simulink model "Localization_Ependorfv2"  (R2025a)
settings: Solver=VariableStepAuto  StartTime=0.0  StopTime=10.0  RelTol=1e-3
libraries: SignalEditorBlockLib x1
settings Model: Creator=Akash  LastModifiedBy=utkar
settings RTWCC: GPUComputeCapability=3.5

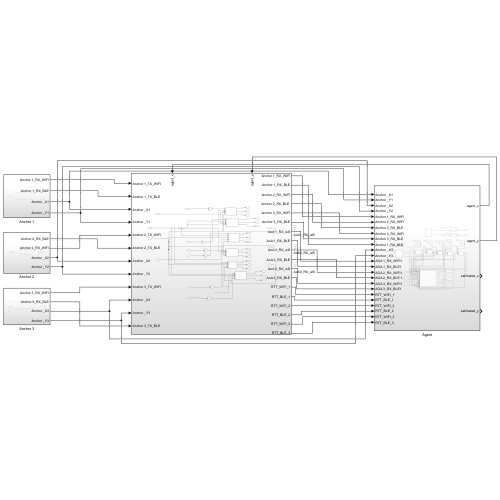
[thumbnail: Simulink's stored preview of the top-level diagram]
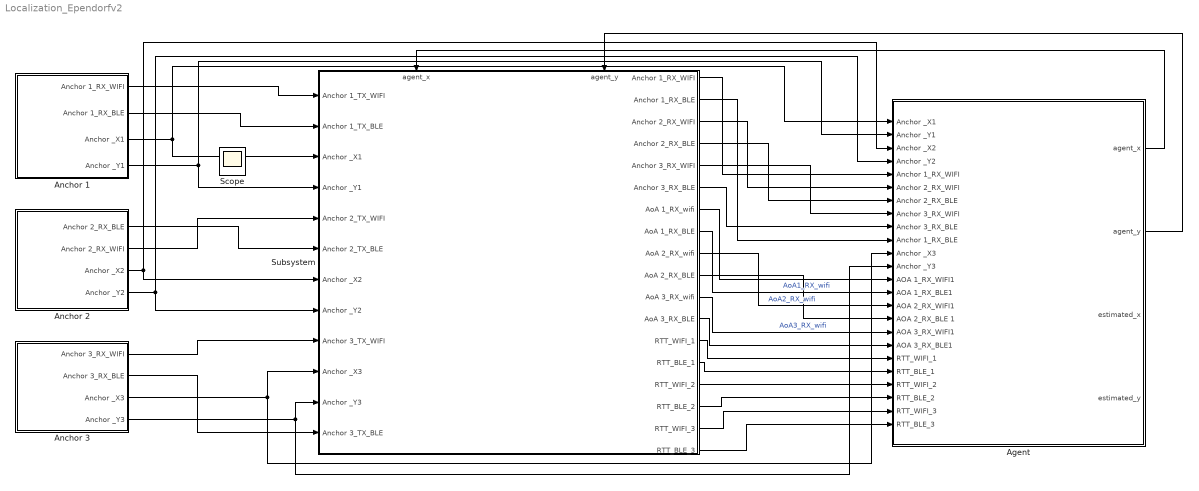
== system Localization_Ependorfv2 ==
  Agent : Subsystem
  Anchor 1 : Subsystem
  Anchor 2 : Subsystem
  Anchor 3 : Subsystem
  Subsystem : Subsystem
      settings: PortSchema="{\"entries\":[{\"content\":{\"sides\":[{\"content\":{\"connectorIds\":[\"In1\",\"In2\",\"In3\",\"In4\",\"In5\",\"In6\",\"In7\",\"In8\",\"In9\",\"In10\",\"In11\",\"In12\"]},\"type\":\"ConnectorPlacement.EquallySpacedRectSide\",\"uuid\":\"0405234f-5b8f-45a1-917e-93d58a1311a8\"},{\"content\":{\"connectorIds\":[\"Out1\",\"Out2\",\"Out3\",\"Out4\",\"Out5\",\"Out6\",\"Out7\",\"Out8\",\"Out9\",\"Out10\",\"Out11\",\"Out12\",\"Out13\",\"Out14\",\"Out15\",\"Out16\",\"Out17\",\"Out18\"],\"side\":\"RIGHT\"},\"type\":\"ConnectorPlacement.EquallySpacedRectSide\",\"uuid\":\"39d2f27a-3797-45c8-9e26-1762cabd752a\"},{\"content\":{\"connectorIds\":[\"In13\",\"In14\"],\"side\":\"TOP\"},\"type\":\"ConnectorPlacement.EquallySpacedRectSide\",\"uuid\":\"f6177108-a7d2-4d89-9cd9-46479219c011\"}]},\"type\":\"ConnectorPlacement.EquallySpacedConnector\",\"uuid\":\"e67eb188-6063-4e30-a59d-3af2b75346f2\"}],\"packageUris\":[\"http://schema.mathworks.com/mf0/Connector/R2020b\"],\"version\":\"1.0\"}"
  Scope : Scope
      settings: ActiveDisplayYMinimum=-0.44035255255063926  ActiveDisplayYMaximum=0.45352039029310781
  wires:
  Anchor 3/1(Anchor 3_RX_WIFI) -> Subsystem/9(Anchor 3_TX_WIFI)
  Anchor 3/2(Anchor 3_RX_BLE) -> Subsystem/12(Anchor 3_TX_BLE)
  Anchor 1/1(Anchor 1_RX_WIFI) -> Subsystem/1(Anchor 1_TX_WIFI)
  Anchor 1/2(Anchor 1_RX_BLE) -> Subsystem/2(Anchor 1_TX_BLE)
  Subsystem/1(Anchor 1_RX_WIFI) -> Agent/5(Anchor 1_RX_WIFI)
  Subsystem/2(Anchor 1_RX_BLE) -> Agent/10(Anchor 1_RX_BLE)
  Subsystem/3(Anchor 2_RX_WIFI) -> Agent/6(Anchor 2_RX_WIFI)
  Subsystem/4("Anchor 2_RX_BLE ") -> Agent/7("Anchor 2_RX_BLE ")
  Subsystem/5(Anchor 3_RX_WIFI) -> Agent/8(Anchor 3_RX_WIFI)
  Subsystem/6(Anchor 3_RX_BLE) -> Agent/9(Anchor 3_RX_BLE)
  Anchor 1/4(Anchor _Y1) -> Subsystem/4(Anchor _Y1), Agent/2(Anchor _Y1)
  Anchor 2/3(Anchor _X2) -> Agent/3(Anchor _X2), Subsystem/7(Anchor _X2)
  Anchor 2/4(Anchor _Y2) -> Agent/4(Anchor _Y2), Subsystem/8(Anchor _Y2)
  Anchor 3/3(Anchor _X3) -> Agent/11(Anchor _X3), Subsystem/10(Anchor _X3)
  Anchor 3/4(Anchor _Y3) -> Agent/12(Anchor _Y3), Subsystem/11(Anchor _Y3)
  Anchor 1/3(Anchor _X1) -> Subsystem/3(Anchor _X1), Agent/1(Anchor _X1)
  Agent/2(agent_y) -> Subsystem/14(agent_y)
  Agent/1(agent_x) -> Subsystem/13(agent_x)
  Subsystem/7(AoA 1_RX_wifi) -> Agent/13(AOA 1_RX_WIFI1)  "AoA1_RX_wifi"
  Subsystem/9(AoA 2_RX_wifi) -> Agent/15(AOA 2_RX_WIFI1)  "AoA2_RX_wifi"
  Subsystem/8(AoA 1_RX_BLE) -> Agent/14(AOA 1_RX_BLE1)
  Subsystem/10(AoA 2_RX_BLE) -> Agent/16(AOA 2_RX_BLE 1)
  Subsystem/11(AoA 3_RX_wifi) -> Agent/17(AOA 3_RX_WIFI1)  "AoA3_RX_wifi"
  Subsystem/12(AoA 3_RX_BLE) -> Agent/18(AOA 3_RX_BLE1)
  Subsystem/13(RTT_WIFI_1) -> Agent/19(RTT_WIFI_1)
  Subsystem/14(RTT_BLE_1) -> Agent/20(RTT_BLE_1)
  Subsystem/15(RTT_WIFI_2) -> Agent/21(RTT_WIFI_2)
  Subsystem/16(RTT_BLE_2) -> Agent/22(RTT_BLE_2)
  Subsystem/17(RTT_WIFI_3) -> Agent/23(RTT_WIFI_3)
  Subsystem/18(RTT_BLE_3) -> Agent/24(RTT_BLE_3)
  Anchor 2/1(Anchor 2_RX_BLE) -> Subsystem/6(Anchor 2_TX_BLE)
  Anchor 2/2(Anchor 2_RX_WIFI) -> Subsystem/5(Anchor 2_TX_WIFI)

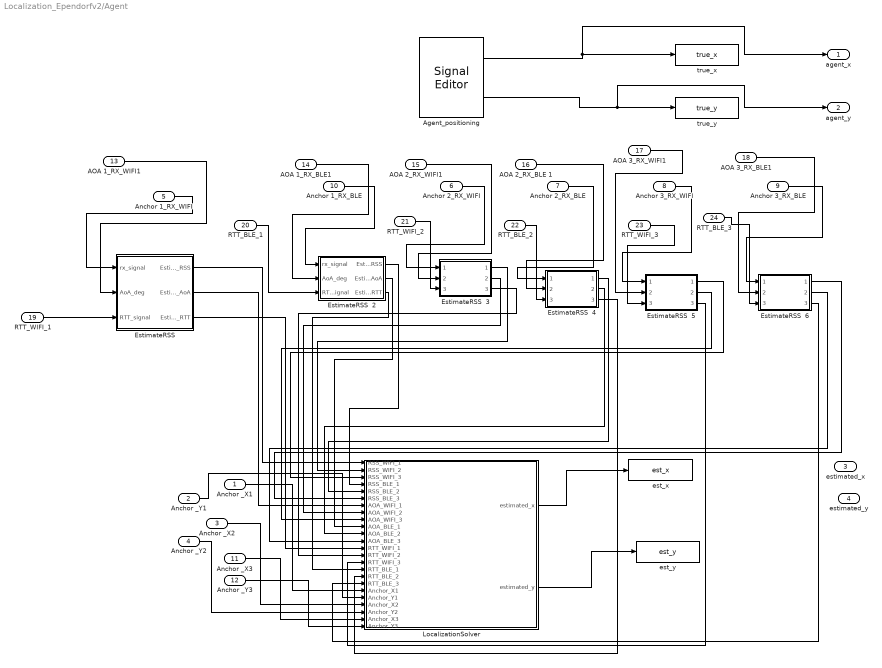
== system Localization_Ependorfv2/Agent ==
  Anchor _X1 : Inport
  Anchor _Y1 : Inport  Port=2
  Anchor _X2 : Inport  Port=3
  Anchor _Y2 : Inport  Port=4
  Anchor 1_RX_WIFI : Inport  Port=5
  Anchor 2_RX_WIFI : Inport  Port=6
  "Anchor 2_RX_BLE " : Inport  Port=7
  Anchor 3_RX_WIFI : Inport  Port=8
  Anchor 3_RX_BLE : Inport  Port=9
  Anchor 1_RX_BLE : Inport  Port=10
  Anchor _X3 : Inport  Port=11
  Anchor _Y3 : Inport  Port=12
  AOA 1_RX_WIFI1 : Inport  Port=13
  AOA 1_RX_BLE1 : Inport  Port=14
  AOA 2_RX_WIFI1 : Inport  Port=15
  AOA 2_RX_BLE 1 : Inport  Port=16
  AOA 3_RX_WIFI1 : Inport  Port=17
  AOA 3_RX_BLE1 : Inport  Port=18
  RTT_WIFI_1 : Inport  Port=19
  RTT_BLE_1 : Inport  Port=20
  RTT_WIFI_2 : Inport  Port=21
  RTT_BLE_2 : Inport  Port=22
  RTT_WIFI_3 : Inport  Port=23
  RTT_BLE_3 : Inport  Port=24
  Agent_positioning : SignalEditorBlockLib/Signal Editor  FileName=agent_path.mat  ActiveScenario=Scenario  ActiveSignal=Agent_x  IsBus=off  OutputBusObjectStr=Bus: BusObject  SampleTime=0  Interpolate=off  ZeroCross=off  OutputAfterFinalValue=Setting to zero  Unit=inherit  PreserveSignalName=on  ApplySigPropsToAllScenarios=on  ApplySigPropsToAllSignals=off  SignalPropertySource=Dialog parameters
  "EstimateRSS " : MATLAB Function  TreatAsAtomicUnit=on
  EstimateRSS  2 : MATLAB Function  TreatAsAtomicUnit=on
  EstimateRSS  3 : MATLAB Function  TreatAsAtomicUnit=on
  EstimateRSS  4 : MATLAB Function  TreatAsAtomicUnit=on
  EstimateRSS  5 : MATLAB Function  TreatAsAtomicUnit=on
  EstimateRSS  6 : MATLAB Function  TreatAsAtomicUnit=on
  LocalizationSolver : MATLAB Function  TreatAsAtomicUnit=on
  est_x : ToWorkspace  VariableName=est_x  SampleTime=-1
  est_y : ToWorkspace  VariableName=est_y  SampleTime=-1
  true_x : ToWorkspace  VariableName=true_x  SampleTime=-1
  true_y : ToWorkspace  VariableName=true_y  SampleTime=-1
  agent_x : Outport
  agent_y : Outport  Port=2
  estimated_x : Outport  Port=3
  estimated_y : Outport  Port=4
  wires:
  LocalizationSolver/2(estimated_y) -> est_y/1
  Anchor 2_RX_WIFI/1 -> EstimateRSS  3/1(rx_signal)
  Anchor 1_RX_BLE/1 -> EstimateRSS  2/1(rx_signal)
  "Anchor 2_RX_BLE "/1 -> EstimateRSS  4/1(rx_signal)
  Anchor 3_RX_WIFI/1 -> EstimateRSS  5/1(rx_signal)
  Anchor 3_RX_BLE/1 -> EstimateRSS  6/1(rx_signal)
  Agent_positioning/1 -> agent_x/1, true_x/1
  Agent_positioning/2 -> agent_y/1, true_y/1
  LocalizationSolver/1(estimated_x) -> est_x/1
  Anchor 1_RX_WIFI/1 -> "EstimateRSS "/1(rx_signal)
  AOA 1_RX_WIFI1/1 -> "EstimateRSS "/2(AoA_deg)
  AOA 1_RX_BLE1/1 -> EstimateRSS  2/2(AoA_deg)
  AOA 2_RX_WIFI1/1 -> EstimateRSS  3/2(AoA_deg)
  AOA 2_RX_BLE 1/1 -> EstimateRSS  4/2(AoA_deg)
  AOA 3_RX_WIFI1/1 -> EstimateRSS  5/2(AoA_deg)
  AOA 3_RX_BLE1/1 -> EstimateRSS  6/2(AoA_deg)
  Anchor _Y3/1 -> LocalizationSolver/24(Anchor_Y3)
  Anchor _X3/1 -> LocalizationSolver/23(Anchor_X3)
  Anchor _Y2/1 -> LocalizationSolver/22(Anchor_Y2)
  Anchor _X2/1 -> LocalizationSolver/21(Anchor_X2)
  Anchor _Y1/1 -> LocalizationSolver/20(Anchor_Y1)
  Anchor _X1/1 -> LocalizationSolver/19(Anchor_X1)
  "EstimateRSS "/1(Estimated_RSS) -> LocalizationSolver/1(RSS_WIFI_1)
  EstimateRSS  3/1(Estimated_RSS) -> LocalizationSolver/2(RSS_WIFI_2)
  EstimateRSS  5/1(Estimated_RSS) -> LocalizationSolver/3(RSS_WIFI_3)
  EstimateRSS  2/1(Estimated_RSS) -> LocalizationSolver/4(RSS_BLE_1)
  EstimateRSS  4/1(Estimated_RSS) -> LocalizationSolver/5(RSS_BLE_2)
  EstimateRSS  6/1(Estimated_RSS) -> LocalizationSolver/6(RSS_BLE_3)
  "EstimateRSS "/2(Estimated_AoA) -> LocalizationSolver/7(AOA_WIFI_1)
  EstimateRSS  3/2(Estimated_AoA) -> LocalizationSolver/8(AOA_WIFI_2)
  EstimateRSS  5/2(Estimated_AoA) -> LocalizationSolver/9(AOA_WIFI_3)
  EstimateRSS  2/2(Estimated_AoA) -> LocalizationSolver/10(AOA_BLE_1)
  EstimateRSS  4/2(Estimated_AoA) -> LocalizationSolver/11(AOA_BLE_2)
  EstimateRSS  6/2(Estimated_AoA) -> LocalizationSolver/12(AOA_BLE_3)
  RTT_WIFI_1/1 -> "EstimateRSS "/3(RTT_signal)
  RTT_BLE_1/1 -> EstimateRSS  2/3(RTT_signal)
  RTT_WIFI_2/1 -> EstimateRSS  3/3(RTT_signal)
  RTT_BLE_2/1 -> EstimateRSS  4/3(RTT_signal)
  RTT_WIFI_3/1 -> EstimateRSS  5/3(RTT_signal)
  RTT_BLE_3/1 -> EstimateRSS  6/3(RTT_signal)
  "EstimateRSS "/3(Estimated_RTT) -> LocalizationSolver/13(RTT_WIFI_1)
  EstimateRSS  2/3(Estimated_RTT) -> LocalizationSolver/16(RTT_BLE_1)
  EstimateRSS  3/3(Estimated_RTT) -> LocalizationSolver/14(RTT_WIFI_2)
  EstimateRSS  4/3(Estimated_RTT) -> LocalizationSolver/17(RTT_BLE_2)
  EstimateRSS  5/3(Estimated_RTT) -> LocalizationSolver/15(RTT_WIFI_3)
  EstimateRSS  6/3(Estimated_RTT) -> LocalizationSolver/18(RTT_BLE_3)

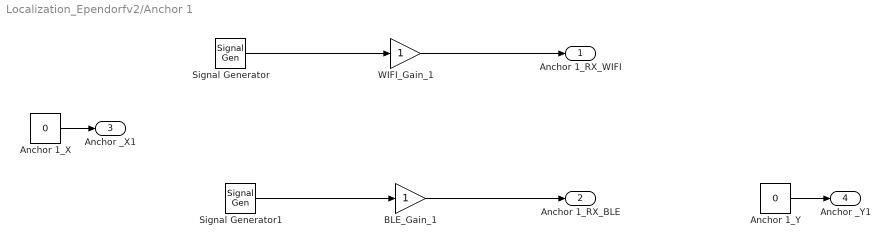
== system Localization_Ependorfv2/Anchor 1 ==
  Anchor 1_X : Constant  Value=0
  Anchor 1_Y : Constant  Value=0
  BLE_Gain_1 : Gain
  Signal Generator : SignalGenerator  Amplitude=10  Units=rad/sec
  Signal Generator1 : SignalGenerator  Amplitude=10  Units=rad/sec
  WIFI_Gain_1 : Gain
  Anchor 1_RX_WIFI : Outport
  Anchor 1_RX_BLE : Outport  Port=2
  Anchor _X1 : Outport  Port=3
  Anchor _Y1 : Outport  Port=4
  wires:
  Signal Generator/1 -> WIFI_Gain_1/1
  Signal Generator1/1 -> BLE_Gain_1/1
  Anchor 1_X/1 -> Anchor _X1/1
  Anchor 1_Y/1 -> Anchor _Y1/1
  WIFI_Gain_1/1 -> Anchor 1_RX_WIFI/1
  BLE_Gain_1/1 -> Anchor 1_RX_BLE/1

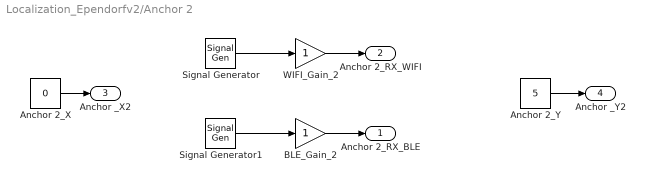
== system Localization_Ependorfv2/Anchor 2 ==
  Anchor 2_X : Constant  Value=0
  Anchor 2_Y : Constant  Value=5
  BLE_Gain_2 : Gain
  Signal Generator : SignalGenerator  Amplitude=10  Units=rad/sec
  Signal Generator1 : SignalGenerator  Amplitude=10  Units=rad/sec
  WIFI_Gain_2 : Gain
  Anchor 2_RX_BLE : Outport
  Anchor 2_RX_WIFI : Outport  Port=2
  Anchor _X2 : Outport  Port=3
  Anchor _Y2 : Outport  Port=4
  wires:
  Signal Generator1/1 -> BLE_Gain_2/1
  Signal Generator/1 -> WIFI_Gain_2/1
  Anchor 2_X/1 -> Anchor _X2/1
  Anchor 2_Y/1 -> Anchor _Y2/1
  WIFI_Gain_2/1 -> Anchor 2_RX_WIFI/1
  BLE_Gain_2/1 -> Anchor 2_RX_BLE/1

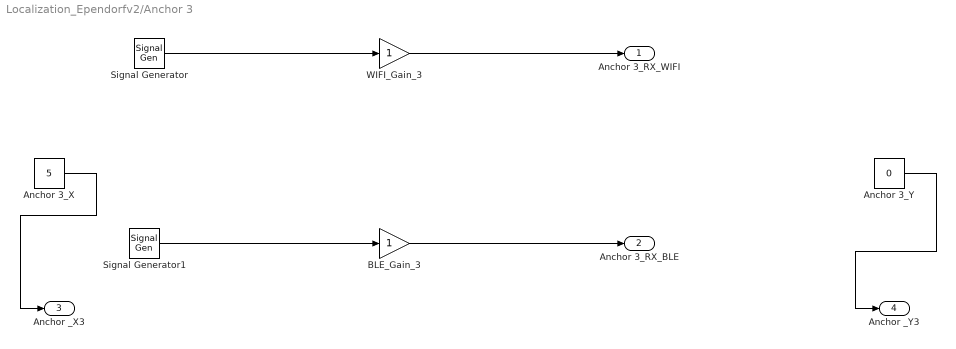
== system Localization_Ependorfv2/Anchor 3 ==
  Anchor 3_X : Constant  Value=5
  Anchor 3_Y : Constant  Value=0
  BLE_Gain_3 : Gain
  Signal Generator : SignalGenerator  Amplitude=10  Units=rad/sec
  Signal Generator1 : SignalGenerator  Amplitude=10  Units=rad/sec
  WIFI_Gain_3 : Gain
  Anchor 3_RX_WIFI : Outport
  Anchor 3_RX_BLE : Outport  Port=2
  Anchor _X3 : Outport  Port=3
  Anchor _Y3 : Outport  Port=4
  wires:
  Signal Generator1/1 -> BLE_Gain_3/1
  Signal Generator/1 -> WIFI_Gain_3/1
  Anchor 3_X/1 -> Anchor _X3/1
  Anchor 3_Y/1 -> Anchor _Y3/1
  WIFI_Gain_3/1 -> Anchor 3_RX_WIFI/1
  BLE_Gain_3/1 -> Anchor 3_RX_BLE/1

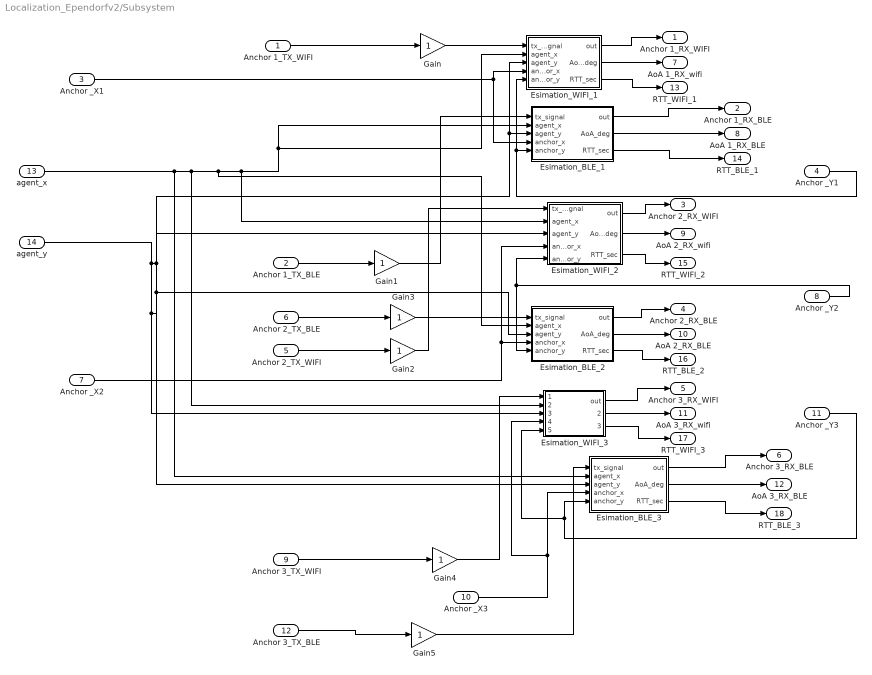
== system Localization_Ependorfv2/Subsystem ==
  Anchor 1_TX_WIFI : Inport
  Anchor 1_TX_BLE : Inport  Port=2
  Anchor _X1 : Inport  Port=3
  Anchor _Y1 : Inport  Port=4
  Anchor 2_TX_WIFI : Inport  Port=5
  Anchor 2_TX_BLE : Inport  Port=6
  Anchor _X2 : Inport  Port=7
  Anchor _Y2 : Inport  Port=8
  Anchor 3_TX_WIFI : Inport  Port=9
  Anchor _X3 : Inport  Port=10
  Anchor _Y3 : Inport  Port=11
  Anchor 3_TX_BLE : Inport  Port=12
  agent_x : Inport  Port=13
  agent_y : Inport  Port=14
  Esimation_BLE_1 : MATLAB Function  TreatAsAtomicUnit=on
  Esimation_BLE_2 : MATLAB Function  TreatAsAtomicUnit=on
  Esimation_BLE_3 : MATLAB Function  TreatAsAtomicUnit=on
  "Esimation_WIFI_1 " : MATLAB Function  TreatAsAtomicUnit=on
  Esimation_WIFI_2 : MATLAB Function  TreatAsAtomicUnit=on
  Esimation_WIFI_3 : MATLAB Function  TreatAsAtomicUnit=on
  Gain{,1..5} (6 alike) : Gain
  Anchor 1_RX_WIFI : Outport
  Anchor 1_RX_BLE : Outport  Port=2
  Anchor 2_RX_WIFI : Outport  Port=3
  "Anchor 2_RX_BLE " : Outport  Port=4
  Anchor 3_RX_WIFI : Outport  Port=5
  Anchor 3_RX_BLE : Outport  Port=6
  AoA 1_RX_wifi : Outport  Port=7
  AoA 1_RX_BLE : Outport  Port=8
  AoA 2_RX_wifi : Outport  Port=9
  AoA 2_RX_BLE : Outport  Port=10
  AoA 3_RX_wifi : Outport  Port=11
  AoA 3_RX_BLE : Outport  Port=12
  RTT_WIFI_1 : Outport  Port=13
  RTT_BLE_1 : Outport  Port=14
  RTT_WIFI_2 : Outport  Port=15
  RTT_BLE_2 : Outport  Port=16
  RTT_WIFI_3 : Outport  Port=17
  RTT_BLE_3 : Outport  Port=18
  wires:
  Anchor 1_TX_WIFI/1 -> Gain/1
  Anchor 1_TX_BLE/1 -> Gain1/1
  Anchor 2_TX_WIFI/1 -> Gain2/1
  Anchor 2_TX_BLE/1 -> Gain3/1
  Anchor 3_TX_WIFI/1 -> Gain4/1
  Anchor 3_TX_BLE/1 -> Gain5/1
  "Esimation_WIFI_1 "/1(out) -> Anchor 1_RX_WIFI/1
  Esimation_BLE_1/1(out) -> Anchor 1_RX_BLE/1
  Esimation_WIFI_2/1(out) -> Anchor 2_RX_WIFI/1
  Esimation_BLE_2/1(out) -> "Anchor 2_RX_BLE "/1
  Esimation_WIFI_3/1(out) -> Anchor 3_RX_WIFI/1
  Esimation_BLE_3/1(out) -> Anchor 3_RX_BLE/1
  Anchor _X3/1 -> Esimation_BLE_3/4(anchor_x), Esimation_WIFI_3/4(anchor_x)
  Gain/1 -> "Esimation_WIFI_1 "/1(tx_signal)
  Gain1/1 -> Esimation_BLE_1/1(tx_signal)
  Gain2/1 -> Esimation_WIFI_2/1(tx_signal)
  Gain3/1 -> Esimation_BLE_2/1(tx_signal)
  Gain4/1 -> Esimation_WIFI_3/1(tx_signal)
  Gain5/1 -> Esimation_BLE_3/1(tx_signal)
  Esimation_BLE_3/2(AoA_deg) -> AoA 3_RX_BLE/1
  Esimation_WIFI_3/2(AoA_deg) -> AoA 3_RX_wifi/1
  Esimation_BLE_2/2(AoA_deg) -> AoA 2_RX_BLE/1
  Esimation_WIFI_2/2(AoA_deg) -> AoA 2_RX_wifi/1
  Esimation_BLE_1/2(AoA_deg) -> AoA 1_RX_BLE/1
  "Esimation_WIFI_1 "/2(AoA_deg) -> AoA 1_RX_wifi/1
  agent_x/1 -> Esimation_BLE_1/2(agent_x), "Esimation_WIFI_1 "/2(agent_x), Esimation_WIFI_2/2(agent_x), Esimation_BLE_2/2(agent_x), Esimation_WIFI_3/2(agent_x), Esimation_BLE_3/2(agent_x)
  agent_y/1 -> Esimation_WIFI_3/3(agent_y), Esimation_BLE_2/3(agent_y), Esimation_WIFI_2/3(agent_y), Esimation_BLE_3/3(agent_y), Esimation_BLE_1/3(agent_y), "Esimation_WIFI_1 "/3(agent_y)
  Anchor _X1/1 -> Esimation_BLE_1/4(anchor_x), "Esimation_WIFI_1 "/4(anchor_x)
  Anchor _Y1/1 -> "Esimation_WIFI_1 "/5(anchor_y), Esimation_BLE_1/5(anchor_y)
  Anchor _X2/1 -> Esimation_BLE_2/4(anchor_x), Esimation_WIFI_2/4(anchor_x)
  Anchor _Y2/1 -> Esimation_BLE_2/5(anchor_y), Esimation_WIFI_2/5(anchor_y)
  Anchor _Y3/1 -> Esimation_WIFI_3/5(anchor_y), Esimation_BLE_3/5(anchor_y)
  "Esimation_WIFI_1 "/3(RTT_sec) -> RTT_WIFI_1/1
  Esimation_BLE_1/3(RTT_sec) -> RTT_BLE_1/1
  Esimation_WIFI_2/3(RTT_sec) -> RTT_WIFI_2/1
  Esimation_BLE_2/3(RTT_sec) -> RTT_BLE_2/1
  Esimation_WIFI_3/3(RTT_sec) -> RTT_WIFI_3/1
  Esimation_BLE_3/3(RTT_sec) -> RTT_BLE_3/1

== matlab function Localization_Ependorfv2/Subsystem/Esimation_BLE_2 ==
  data: tx_signal input; agent_x input; out output; agent_y input; anchor_x input; anchor_y input; AoA_deg output; RTT_sec output
function [out, AoA_deg, RTT_sec] = applyPathLossWithAOA_BLE(tx_signal, agent_x, agent_y, anchor_x, anchor_y)
% applyPathLossWithAOA_BLE: Simulates signal attenuation, AoA, and RTT for BLE

% === 1. Compute Distance ===
d = sqrt((agent_x - anchor_x)^2 + (agent_y - anchor_y)^2);
d0 = 1;
d = max(d, d0);

% === 2. Path Loss Model (BLE)
Ptx = 0;       
PL0 = 50;      % BLE generally has higher base loss
n   = 3;       % Stronger attenuation indoors for BLE
PL  = PL0 + 10 * n * log10(d / d0);

% === 3. Attenuate Signal ===
attenuation = 10.^(-PL / 20);  
out = tx_signal * attenuation;

% === 4. AoA Calculation (BLE - slightly noisier)
aoa_noise_std_deg = 5;
dx = agent_x - anchor_x;
dy = agent_y - anchor_y;
AoA_rad = atan2(dy, dx);
AoA_rad_noisy = AoA_rad + deg2rad(randn * aoa_noise_std_deg);
AoA_deg = mod(rad2deg(AoA_rad_noisy), 360);

% === 5. Simulate RTT (BLE less accurate: ~5 ns noise)
c = 3e8;  
rtt_noise_std = 5e-9;  
RTT_sec = 2 * d / c + randn * rtt_noise_std;

end

== matlab function Localization_Ependorfv2/Subsystem/Esimation_WIFI_3 ==
  data: tx_signal input; agent_x input; out output; agent_y input; anchor_x input; anchor_y input; AoA_deg output; RTT_sec output
function [out, AoA_deg, RTT_sec] = applyPathLossWithAOA_WiFi(tx_signal, agent_x, agent_y, anchor_x, anchor_y)
% applyPathLossWithAOA_WiFi: Simulates signal attenuation, AoA, and RTT for WiFi

% === 1. Compute Distance ===
d = sqrt((agent_x - anchor_x)^2 + (agent_y - anchor_y)^2);
d0 = 1;
d = max(d, d0);

% === 2. Path Loss Model (WiFi) ===
Ptx = 0;       % dBm
PL0 = 30;      % Reference loss at 1m (WiFi)
n   = 2.2;     % Path loss exponent for indoor WiFi
PL  = PL0 + 10 * n * log10(d / d0);

% === 3. Attenuate Signal ===
attenuation = 10.^(-PL / 20);  
out = tx_signal * attenuation;

% === 4. AoA Calculation (WiFi - lower noise)
aoa_noise_std_deg = 2;
dx = agent_x - anchor_x;
dy = agent_y - anchor_y;
AoA_rad = atan2(dy, dx);
AoA_rad_noisy = AoA_rad + deg2rad(randn * aoa_noise_std_deg);
AoA_deg = mod(rad2deg(AoA_rad_noisy), 360);

% === 5. Simulate RTT (WiFi typically accurate to ~1 ns)
c = 3e8;  
rtt_noise_std = 1e-9;  
RTT_sec = 2 * d / c + randn * rtt_noise_std;

end

== matlab function Localization_Ependorfv2/Subsystem/Esimation_BLE_3 ==
  data: tx_signal input; agent_x input; agent_y input; out output; anchor_x input; anchor_y input; AoA_deg output; RTT_sec output
function [out, AoA_deg, RTT_sec] = applyPathLossWithAOA_BLE(tx_signal, agent_x, agent_y, anchor_x, anchor_y)
% applyPathLossWithAOA_BLE: Simulates signal attenuation, AoA, and RTT for BLE

% === 1. Compute Distance ===
d = sqrt((agent_x - anchor_x)^2 + (agent_y - anchor_y)^2);
d0 = 1;
d = max(d, d0);

% === 2. Path Loss Model (BLE)
Ptx = 0;       
PL0 = 50;      % BLE generally has higher base loss
n   = 3;       % Stronger attenuation indoors for BLE
PL  = PL0 + 10 * n * log10(d / d0);

% === 3. Attenuate Signal ===
attenuation = 10.^(-PL / 20);  
out = tx_signal * attenuation;

% === 4. AoA Calculation (BLE - slightly noisier)
aoa_noise_std_deg = 5;
dx = agent_x - anchor_x;
dy = agent_y - anchor_y;
AoA_rad = atan2(dy, dx);
AoA_rad_noisy = AoA_rad + deg2rad(randn * aoa_noise_std_deg);
AoA_deg = mod(rad2deg(AoA_rad_noisy), 360);

% === 5. Simulate RTT (BLE less accurate: ~5 ns noise)
c = 3e8;  
rtt_noise_std = 5e-9;  
RTT_sec = 2 * d / c + randn * rtt_noise_std;

end

== matlab function Localization_Ependorfv2/Agent/LocalizationSolver ==
  data: RSS_WIFI_1 input; RSS_WIFI_2 input; RSS_WIFI_3 input; estimated_x output double size=1; estimated_y output double size=1; RSS_BLE_1 input double size=1; RSS_BLE_2 input double size=1; RSS_BLE_3 input; AOA_WIFI_1 input; AOA_WIFI_2 input; AOA_WIFI_3 input; AOA_BLE_1 input; AOA_BLE_2 input; AOA_BLE_3 input; RTT_WIFI_1 input; RTT_WIFI_2 input; RTT_WIFI_3 input; RTT_BLE_1 input; RTT_BLE_2 input; RTT_BLE_3 input; Anchor_X1 input double size=1; Anchor_Y1 input double size=1; Anchor_X2 input double size=1; Anchor_Y2 input double size=1; Anchor_X3 input double size=1; Anchor_Y3 input double size=1
function [estimated_x, estimated_y] = fcn( ...
    RSS_WIFI_1, RSS_WIFI_2, RSS_WIFI_3, ...
    RSS_BLE_1,  RSS_BLE_2,  RSS_BLE_3, ...
    AOA_WIFI_1, AOA_WIFI_2, AOA_WIFI_3, ...
    AOA_BLE_1,  AOA_BLE_2,  AOA_BLE_3, ...
    RTT_WIFI_1, RTT_WIFI_2, RTT_WIFI_3, ...
    RTT_BLE_1,  RTT_BLE_2,  RTT_BLE_3, ...
    Anchor_X1, Anchor_Y1, ...
    Anchor_X2, Anchor_Y2, ...
    Anchor_X3, Anchor_Y3)

% === 1. Collect RSS measurements ===
RSS_wifi = [RSS_WIFI_1; RSS_WIFI_2; RSS_WIFI_3];
RSS_ble  = [RSS_BLE_1;  RSS_BLE_2;  RSS_BLE_3];
RSS_all  = [RSS_wifi; RSS_ble];

% === 2. Anchor positions duplicated for BLE ===
anchors_x = [Anchor_X1; Anchor_X2; Anchor_X3];
anchors_y = [Anchor_Y1; Anchor_Y2; Anchor_Y3];
anchors_x_all = [anchors_x; anchors_x];  % Wi-Fi + BLE
anchors_y_all = [anchors_y; anchors_y];

% === 3. Convert RSS to distance ===
Pt  = 0;    % Transmit power [dBm]
PL0 = 44;   % Path loss at 1m [dB]
n   = 1.9;  % Path loss exponent
d0  = 1;    % reference distance [m]

estimated_d_rss = d0 * 10.^((Pt - PL0 - RSS_all) ./ (10 * n));
estimated_d_rss = min(estimated_d_rss, 100); % cap large distances

% === 4. Combine all AoA angles ===
aoa_angles_deg = [AOA_WIFI_1; AOA_WIFI_2; AOA_WIFI_3; ...
                  AOA_BLE_1;  AOA_BLE_2;  AOA_BLE_3];

% === 5. RTT-based Distance Estimation ===
c = 3e8;  % speed of light [m/s]
RTT_all = [RTT_WIFI_1; RTT_WIFI_2; RTT_WIFI_3; ...
           RTT_BLE_1;  RTT_BLE_2;  RTT_BLE_3];
estimated_d_rtt = RTT_all * c / 2;
estimated_d_rtt = min(estimated_d_rtt, 100); 

% === 6. Initial Guess ===
persistent last_est
if isempty(last_est)
    last_est = [mean(anchors_x_all), mean(anchors_y_all)];
end
x0 = last_est(1);
y0 = last_est(2);

% === 7. Optimization using RSS + AoA + RTT ===
options = optimset('Display','off');
estimated_pos = fminsearch( ...
    @(p) objective(p, anchors_x_all, anchors_y_all, ...
                   estimated_d_rss, aoa_angles_deg, ...
                   anchors_x_all, anchors_y_all, estimated_d_rtt), ...
    [x0, y0], options);

% === 8. Output ===
estimated_x = estimated_pos(1);
estimated_y = estimated_pos(2);

% === 9. Save estimate ===
last_est = estimated_pos;

end

% === Objective Function: RSS + AoA + RTT ===
function err = objective(p, anchors_x, anchors_y, estimated_d_rss, ...
                         aoa_angles_deg, rtt_x, rtt_y, estimated_d_rtt)
    x = p(1);
    y = p(2);

    % RSS Distance Error
    distances_rss = sqrt((anchors_x - x).^2 + (anchors_y - y).^2);
    dist_error = sum((distances_rss - estimated_d_rss).^2);

    % AoA Error
    angle_error = 0;
    for i = 1:length(anchors_x)
        dx = x - anchors_x(i);
        dy = y - anchors_y(i);
        est_angle = mod(rad2deg(atan2(dy, dx)), 360);
        true_angle = aoa_angles_deg(i);
        diff_angle = abs(est_angle - true_angle);
        diff_angle = min(diff_angle, 360 - diff_angle);  % shortest angle
        angle_error = angle_error + diff_angle^2;
    end

    % RTT Distance Error
    distances_rtt = sqrt((rtt_x - x).^2 + (rtt_y - y).^2);
    rtt_error = sum((distances_rtt - estimated_d_rtt).^2);

    % Total error (tune weights if needed)
    err = 1.0 * dist_error + 0.5 * angle_error + 0.5 * rtt_error;
end

== matlab function Localization_Ependorfv2/Agent/EstimateRSS  3 ==
  data: rx_signal input; Estimated_RSS output; AoA_deg input; Estimated_AoA output; RTT_signal input; Estimated_RTT output
function [Estimated_RSS, Estimated_AoA, Estimated_RTT] = EstimateRSSAOARTT(rx_signal, AoA_deg, RTT_signal)
%#codegen
% Estimates RSS, AoA, and RTT from received signals

% === 1. Estimate RSS ===
power = rx_signal .^ 2;
power(power < 1e-12) = 1e-12;
Estimated_RSS = 10 * log10(power / 1e-3);
Estimated_RSS = Estimated_RSS + 1.5 * randn(size(rx_signal));  % RSS noise
Estimated_RSS = max(min(Estimated_RSS, 0), -100);              % clamp

% === 2. Estimate AoA ===
Estimated_AoA = mod(AoA_deg + 2.0 * randn(), 360);             % AoA noise

% === 3. Estimate RTT-based Distance ===
c = 3e8; % Speed of light
RTT_noise = 2e-9 * randn();  % 2 ns noise (~0.6m)
Estimated_RTT = RTT_signal + RTT_noise; % one-way range

== matlab function Localization_Ependorfv2/Agent/EstimateRSS  ==
  data: rx_signal input; Estimated_RSS output; AoA_deg input; Estimated_AoA output; RTT_signal input; Estimated_RTT output
function [Estimated_RSS, Estimated_AoA, Estimated_RTT] = EstimateRSSAOARTT(rx_signal, AoA_deg, RTT_signal)
%#codegen
% Estimates RSS, AoA, and RTT from received signals

% === 1. Estimate RSS ===
power = rx_signal .^ 2;
power(power < 1e-12) = 1e-12;
Estimated_RSS = 10 * log10(power / 1e-3);
Estimated_RSS = Estimated_RSS + 1.5 * randn(size(rx_signal));  % RSS noise
Estimated_RSS = max(min(Estimated_RSS, 0), -100);              % clamp

% === 2. Estimate AoA ===
Estimated_AoA = mod(AoA_deg + 2.0 * randn(), 360);             % AoA noise

% === 3. Estimate RTT-based Distance ===
c = 3e8; % Speed of light
RTT_noise = 2e-9 * randn();  % 2 ns noise (~0.6m)
Estimated_RTT = RTT_signal + RTT_noise; % one-way range

== matlab function Localization_Ependorfv2/Agent/EstimateRSS  2 ==
  data: rx_signal input; Estimated_RSS output; AoA_deg input; Estimated_AoA output; RTT_signal input; Estimated_RTT output
function [Estimated_RSS, Estimated_AoA, Estimated_RTT] = EstimateRSSAOARTT(rx_signal, AoA_deg, RTT_signal)
%#codegen
% Estimates RSS, AoA, and RTT from received signals

% === 1. Estimate RSS ===
power = rx_signal .^ 2;
power(power < 1e-12) = 1e-12;
Estimated_RSS = 10 * log10(power / 1e-3);
Estimated_RSS = Estimated_RSS + 1.5 * randn(size(rx_signal));  % RSS noise
Estimated_RSS = max(min(Estimated_RSS, 0), -100);              % clamp

% === 2. Estimate AoA ===
Estimated_AoA = mod(AoA_deg + 2.0 * randn(), 360);             % AoA noise

% === 3. Estimate RTT-based Distance ===
c = 3e8; % Speed of light
RTT_noise = 2e-9 * randn();  % 2 ns noise (~0.6m)
Estimated_RTT = RTT_signal + RTT_noise; % one-way range

== matlab function Localization_Ependorfv2/Agent/EstimateRSS  6 ==
  data: rx_signal input; Estimated_RSS output; AoA_deg input; Estimated_AoA output; RTT_signal input; Estimated_RTT output
function [Estimated_RSS, Estimated_AoA, Estimated_RTT] = EstimateRSSAOARTT(rx_signal, AoA_deg, RTT_signal)
%#codegen
% Estimates RSS, AoA, and RTT from received signals

% === 1. Estimate RSS ===
power = rx_signal .^ 2;
power(power < 1e-12) = 1e-12;
Estimated_RSS = 10 * log10(power / 1e-3);
Estimated_RSS = Estimated_RSS + 1.5 * randn(size(rx_signal));  % RSS noise
Estimated_RSS = max(min(Estimated_RSS, 0), -100);              % clamp

% === 2. Estimate AoA ===
Estimated_AoA = mod(AoA_deg + 2.0 * randn(), 360);             % AoA noise

% === 3. Estimate RTT-based Distance ===
c = 3e8; % Speed of light
RTT_noise = 2e-9 * randn();  % 2 ns noise (~0.6m)
Estimated_RTT = RTT_signal + RTT_noise; % one-way range

== matlab function Localization_Ependorfv2/Agent/EstimateRSS  5 ==
  data: rx_signal input; Estimated_RSS output; AoA_deg input; Estimated_AoA output; RTT_signal input; Estimated_RTT output
function [Estimated_RSS, Estimated_AoA, Estimated_RTT] = EstimateRSSAOARTT(rx_signal, AoA_deg, RTT_signal)
%#codegen
% Estimates RSS, AoA, and RTT from received signals

% === 1. Estimate RSS ===
power = rx_signal .^ 2;
power(power < 1e-12) = 1e-12;
Estimated_RSS = 10 * log10(power / 1e-3);
Estimated_RSS = Estimated_RSS + 1.5 * randn(size(rx_signal));  % RSS noise
Estimated_RSS = max(min(Estimated_RSS, 0), -100);              % clamp

% === 2. Estimate AoA ===
Estimated_AoA = mod(AoA_deg + 2.0 * randn(), 360);             % AoA noise

% === 3. Estimate RTT-based Distance ===
c = 3e8; % Speed of light
RTT_noise = 2e-9 * randn();  % 2 ns noise (~0.6m)
Estimated_RTT = RTT_signal + RTT_noise; % one-way range

== matlab function Localization_Ependorfv2/Agent/EstimateRSS  4 ==
  data: rx_signal input; Estimated_RSS output; AoA_deg input; Estimated_AoA output; RTT_signal input; Estimated_RTT output
function [Estimated_RSS, Estimated_AoA, Estimated_RTT] = EstimateRSSAOARTT(rx_signal, AoA_deg, RTT_signal)
%#codegen
% Estimates RSS, AoA, and RTT from received signals

% === 1. Estimate RSS ===
power = rx_signal .^ 2;
power(power < 1e-12) = 1e-12;
Estimated_RSS = 10 * log10(power / 1e-3);
Estimated_RSS = Estimated_RSS + 1.5 * randn(size(rx_signal));  % RSS noise
Estimated_RSS = max(min(Estimated_RSS, 0), -100);              % clamp

% === 2. Estimate AoA ===
Estimated_AoA = mod(AoA_deg + 2.0 * randn(), 360);             % AoA noise

% === 3. Estimate RTT-based Distance ===
c = 3e8; % Speed of light
RTT_noise = 2e-9 * randn();  % 2 ns noise (~0.6m)
Estimated_RTT = RTT_signal + RTT_noise; % one-way range

== matlab function Localization_Ependorfv2/Subsystem/Esimation_BLE_1 ==
  data: tx_signal input; agent_x input; agent_y input; out output; anchor_x input; anchor_y input; AoA_deg output; RTT_sec output
function [out, AoA_deg, RTT_sec] = applyPathLossWithAOA_BLE(tx_signal, agent_x, agent_y, anchor_x, anchor_y)
% applyPathLossWithAOA_BLE: Simulates signal attenuation, AoA, and RTT for BLE

% === 1. Compute Distance ===
d = sqrt((agent_x - anchor_x)^2 + (agent_y - anchor_y)^2);
d0 = 1;
d = max(d, d0);

% === 2. Path Loss Model (BLE)
Ptx = 0;       
PL0 = 50;      % BLE generally has higher base loss
n   = 3;       % Stronger attenuation indoors for BLE
PL  = PL0 + 10 * n * log10(d / d0);

% === 3. Attenuate Signal ===
attenuation = 10.^(-PL / 20);  
out = tx_signal * attenuation;

% === 4. AoA Calculation (BLE - slightly noisier)
aoa_noise_std_deg = 5;
dx = agent_x - anchor_x;
dy = agent_y - anchor_y;
AoA_rad = atan2(dy, dx);
AoA_rad_noisy = AoA_rad + deg2rad(randn * aoa_noise_std_deg);
AoA_deg = mod(rad2deg(AoA_rad_noisy), 360);

% === 5. Simulate RTT (BLE less accurate: ~5 ns noise)
c = 3e8;  
rtt_noise_std = 5e-9;  
RTT_sec = 2 * d / c + randn * rtt_noise_std;

end

== matlab function Localization_Ependorfv2/Subsystem/Esimation_WIFI_1  ==
  data: tx_signal input; agent_x input; agent_y input; anchor_x input; anchor_y input; out output; AoA_deg output; RTT_sec output
function [out, AoA_deg, RTT_sec] = applyPathLossWithAOA_WiFi(tx_signal, agent_x, agent_y, anchor_x, anchor_y)
% applyPathLossWithAOA_WiFi: Simulates signal attenuation, AoA, and RTT for WiFi

% === 1. Compute Distance ===
d = sqrt((agent_x - anchor_x)^2 + (agent_y - anchor_y)^2);
d0 = 1;
d = max(d, d0);

% === 2. Path Loss Model (WiFi) ===
Ptx = 0;       % dBm
PL0 = 30;      % Reference loss at 1m (WiFi)
n   = 2.2;     % Path loss exponent for indoor WiFi
PL  = PL0 + 10 * n * log10(d / d0);

% === 3. Attenuate Signal ===
attenuation = 10.^(-PL / 20);  
out = tx_signal * attenuation;

% === 4. AoA Calculation (WiFi - lower noise)
aoa_noise_std_deg = 2;
dx = agent_x - anchor_x;
dy = agent_y - anchor_y;
AoA_rad = atan2(dy, dx);
AoA_rad_noisy = AoA_rad + deg2rad(randn * aoa_noise_std_deg);
AoA_deg = mod(rad2deg(AoA_rad_noisy), 360);

% === 5. Simulate RTT (WiFi typically accurate to ~1 ns)
c = 3e8;  
rtt_noise_std = 1e-9;  
RTT_sec = 2 * d / c + randn * rtt_noise_std;

end

== matlab function Localization_Ependorfv2/Subsystem/Esimation_WIFI_2 ==
  data: tx_signal input; agent_x input; agent_y input; out output; anchor_x input; anchor_y input; AoA_deg output; RTT_sec output
function [out, AoA_deg, RTT_sec] = applyPathLossWithAOA_WiFi(tx_signal, agent_x, agent_y, anchor_x, anchor_y)
% applyPathLossWithAOA_WiFi: Simulates signal attenuation, AoA, and RTT for WiFi

% === 1. Compute Distance ===
d = sqrt((agent_x - anchor_x)^2 + (agent_y - anchor_y)^2);
d0 = 1;
d = max(d, d0);

% === 2. Path Loss Model (WiFi) ===
Ptx = 0;       % dBm
PL0 = 30;      % Reference loss at 1m (WiFi)
n   = 2.2;     % Path loss exponent for indoor WiFi
PL  = PL0 + 10 * n * log10(d / d0);

% === 3. Attenuate Signal ===
attenuation = 10.^(-PL / 20);  
out = tx_signal * attenuation;

% === 4. AoA Calculation (WiFi - lower noise)
aoa_noise_std_deg = 2;
dx = agent_x - anchor_x;
dy = agent_y - anchor_y;
AoA_rad = atan2(dy, dx);
AoA_rad_noisy = AoA_rad + deg2rad(randn * aoa_noise_std_deg);
AoA_deg = mod(rad2deg(AoA_rad_noisy), 360);

% === 5. Simulate RTT (WiFi typically accurate to ~1 ns)
c = 3e8;  
rtt_noise_std = 1e-9;  
RTT_sec = 2 * d / c + randn * rtt_noise_std;

end
